simulink model "radia_nonlinear_reactor"  (R2026a)
settings: Solver=FixedStepDiscrete  StopTime=0.1  FixedStep=radia_nonlinear_reactor_config.sample_time_s
model workspace (MAT data in the model file):
  radia_nonlinear_reactor_config.schema = 'radia.simulink.nonlinear-hdiv-mmm-reactor.v1'
  radia_nonlinear_reactor_config.backend = 'matlab-level2+radia-mex-handle'
  radia_nonlinear_reactor_config.source = 'toroidal-hdiv-mmm-mode'
  radia_nonlinear_reactor_config.python_per_step = 0
  radia_nonlinear_reactor_config.n_modes = 1
  radia_nonlinear_reactor_config.n_samples = 288
  radia_nonlinear_reactor_config.demag_row_major = 0
  radia_nonlinear_reactor_config.magnetization_modes_row_major = [0 0.93606553498 0 -0.8106565329 0.46803276749 0 -0.8106565329 -0.46803276749 0 -1.14634966121e-16 -0.93606553498 0 ... (864 elements, 1x864)]
  radia_nonlinear_reactor_config.sample_weights = [3.6610107354e-07 3.6610107354e-07 3.6610107354e-07 3.6610107354e-07 3.6610107354e-07 3.6610107354e-07 3.59829327123e-07 3.59829327123e-07 3.59829327123e-07 3.59829327123e-07 3.59829327123e-07 3.59829327123e-07 ... (288 elements, 288x1)]
  radia_nonlinear_reactor_config.sample_points_m = [0.0534150635095 0.0267075317547 -0.0267075317547 -0.0534150635095 -0.0267075317547 0.0267075317547 0.0525 0.02625 -0.02625 -0.0525 -0.02625 0.02625 ... (864 elements, 288x3)]
  radia_nonlinear_reactor_config.excitation_per_amp = 0.025389141824
  radia_nonlinear_reactor_config.bh_curve_H_A_per_m_B_T = [0  0; 50  0.55; 100  0.95; 200  1.3; 500  1.55; 1000  1.68; 2000  1.78; 5000  1.9; 10000  1.98; 50000  2.08; 200000  2.28]
  radia_nonlinear_reactor_config.magnetization_table_A_per_m = [0; 437626.093503; 755885.979687; 1034307.1301; 1232950.80896; 1335901.52197; 1414478.99352; 1506971.95937; 1565633.93661; 1605211.40816; 1614366.35125]
  radia_nonlinear_reactor_config.field_table_A_per_m = [0; 50; 100; 200; 500; 1000; 2000; 5000; 10000; 50000; 200000]
  radia_nonlinear_reactor_config.air_inductance_H = 8.12452538369e-06
  radia_nonlinear_reactor_config.winding_resistance_Ohm = 0.3
  radia_nonlinear_reactor_config.sample_time_s = 0.0001
  radia_nonlinear_reactor_config.initial_current_A = 0
  radia_nonlinear_reactor_config.residual_tolerance = 1e-09
  radia_nonlinear_reactor_config.max_iterations = 40
  radia_nonlinear_reactor_config.line_search_minimum = 9.53674316406e-07
  radia_nonlinear_reactor_config.flux_linkage_definition = "lambda=L_air*i+mu0*excitation_per_amp'*magnetization"
  radia_nonlinear_reactor_config.voltage_definition = "v=R*i+(lambda-lambda_previous)/dt"
  radia_nonlinear_reactor_config.field_output = "sampled B magnitude in tesla"
  radia_nonlinear_reactor_config.geometry.kind = "toroid"
  radia_nonlinear_reactor_config.geometry.major_radius_m = 0.05
  radia_nonlinear_reactor_config.geometry.minor_radius_m = 0.01
  radia_nonlinear_reactor_config.geometry.turns = 80
libraries: radia_simulink_library x2
settings Model: Creator=Administrator  LastModifiedBy=Administrator

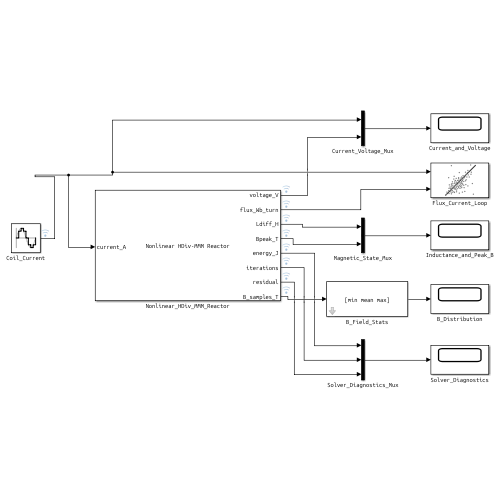
[thumbnail: Simulink's stored preview of the top-level diagram]
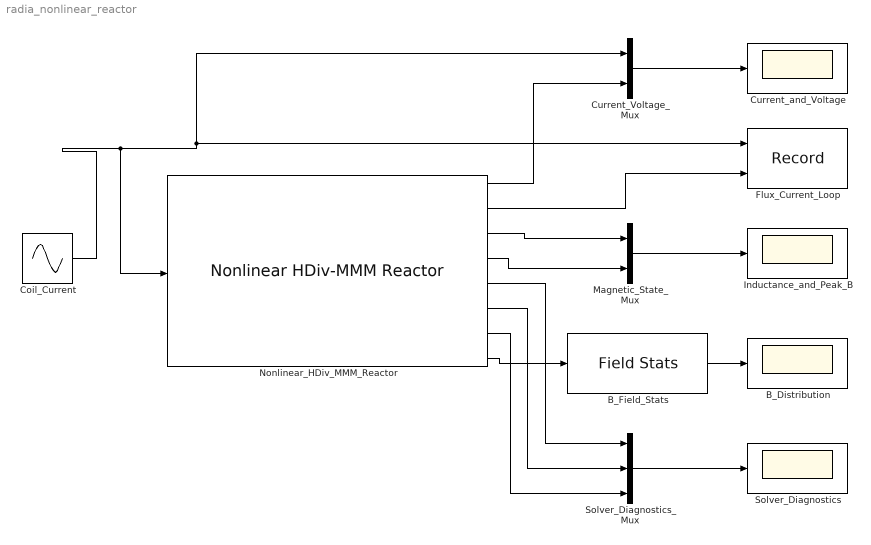
== system radia_nonlinear_reactor ==
  B_Distribution : Scope
  B_Field_Stats : radia_simulink_library/Utilities/Field Stats  Tag=RadiaFieldStats
  Coil_Current : Sin  Amplitude=20  Frequency=2*pi*50  SampleTime=radia_nonlinear_reactor_config.sample_time_s
  Current_Voltage_Mux : Mux  Inputs=2
  Current_and_Voltage : Scope
  Flux_Current_Loop : Record  NumPorts=2.0  FileSettingsInternal="{\"entries\":[{\"content\":{\"excelSettings\":{\"content\":{},\"type\":\"Streamout.ExcelSettings\"},\"parquetSettings\":{\"content\":{},\"type\":\"Streamout.ParquetSettings\"}},\"type\":\"Streamout.FileSettingStorage\",\"uuid\":\"\"}],\"packageUris\":[\"http:\\/\\/schema.mathworks.com\\/mf0\\/streamout_blocks\\/R2020a\"],\"version\":\"1.0\"}"  FrameSettings=[0, 0]  Layout=[1 1]  SignalsInternal="{\"entries\":[{\"content\":{\"signals\":[{\"content\":{\"blockPath\":[],\"dimensions\":[1],\"domain\":\"\",\"lineColor\":\"#a2142f\",\"plots\":[ 1 ],\"port\":1,\"signalID\":1,\"signalName\":\"current_A\"},\"type\":\"RecordBlkView.Signal\",\"uuid\":\"\"},{\"content\":{\"blockPath\":[],\"dimensions\":[1],\"domain\":\"\",\"lineColor\":\"#139fff\",\"plots\":[ 1 ],\"port\":2,\"signalID\":2,\"signalName\":\"flux_Wb_turn\"},\"type\":\"RecordBlkView.Signal\",\"uuid\":\"\"}]},\"type\":\"RecordBlkView.InputSignals\",\"uuid\":\"\"}],\"packageUris\":[\"http:\\/\\/schema.mathworks.com\\/mf0\\/streamout_blocks\\/R2020a\"],\"version\":\"1.0\"}"  VisualizationBindings="{\"xyplotplugin\":{\"info\":[{\"series\":[{\"bindingParametersList\":[{\"parameter\":\"X-Axis\",\"signalID\":1,\"signalName\":\"current_A\"},{\"parameter\":\"Y-Axis\",\"signalID\":2,\"signalName\":\"flux_Wb_turn\"}],\"seriesID\":0}],\"subplotID\":1}]}}"  CompatibilityTag=XY  st=-1
  Inductance_and_Peak_B : Scope
  Magnetic_State_Mux : Mux  Inputs=2
  Nonlinear_HDiv_MMM_Reactor : radia_simulink_library/Reduced Models/Nonlinear HDiv-MMM Reactor  reactor_config=radia_nonlinear_reactor_config
      settings: SourceProductName=Radia
  Solver_Diagnostics : Scope
  Solver_Diagnostics_Mux : Mux  Inputs=3
  wires:
  Coil_Current/1 -> Current_Voltage_Mux/1, Flux_Current_Loop/1, Nonlinear_HDiv_MMM_Reactor/1
  Nonlinear_HDiv_MMM_Reactor/1 -> Current_Voltage_Mux/2
  Nonlinear_HDiv_MMM_Reactor/2 -> Flux_Current_Loop/2
  Nonlinear_HDiv_MMM_Reactor/3 -> Magnetic_State_Mux/1
  Nonlinear_HDiv_MMM_Reactor/4 -> Magnetic_State_Mux/2
  Nonlinear_HDiv_MMM_Reactor/5 -> Solver_Diagnostics_Mux/1
  Nonlinear_HDiv_MMM_Reactor/6 -> Solver_Diagnostics_Mux/2
  Nonlinear_HDiv_MMM_Reactor/7 -> Solver_Diagnostics_Mux/3
  Nonlinear_HDiv_MMM_Reactor/8 -> B_Field_Stats/1
  Current_Voltage_Mux/1 -> Current_and_Voltage/1
  Magnetic_State_Mux/1 -> Inductance_and_Peak_B/1
  B_Field_Stats/1 -> B_Distribution/1
  Solver_Diagnostics_Mux/1 -> Solver_Diagnostics/1
